simulink library "control_lib"  (R2022b)
settings: Solver=ode45  StartTime=0.0  StopTime=10.0  RelTol=1e-3
settings Model: Creator=nicholas  LastModifiedBy=bensweet
settings SolverCC: AlgebraicLoopSolver=TrustRegion
settings DataIOCC: LimitDataPoints=on  SaveFormat=Array  SignalLoggingSaveFormat=ModelDataLogs  ReturnWorkspaceOutputs=off
settings OptimizationCC: BlockReduction=off  BooleanDataType=off  ExpressionDepthLimit=2147483647  LifeSpan=inf
settings DebuggingCC: SaveWithParameterizedLinksMsg=none  UnderspecifiedInitializationDetection=Classic  MergeDetectMultiDrivingBlocksExec=none  SignalResolutionControl=TryResolveAllWithWarning  UnconnectedInputMsg=warning  UnconnectedOutputMsg=warning  UnconnectedLineMsg=warning  AllowSymbolicDim=off  StateNameClashWarn=warning  PregeneratedLibrarySubsystemCodeDiagnostic=none  SFUnexpectedBacktrackingDiag=warning  SFNoUnconditionalDefaultTransitionDiag=warning  SFExecutionAtInitializationDiag=none  SFMachineParentedDataDiag=warning  ArithmeticOperatorsInVariantConditions=warning
settings HardwareCC: ProdBitPerPointer=32  ProdBitPerSizeT=32  ProdBitPerPtrDiffT=32  ProdLargestAtomicFloat=None  ProdIntDivRoundTo=Undefined  ProdEndianess=Unspecified  ProdWordSize=32  ProdHWDeviceType=32-bit Generic  TargetUnknown=on
settings ModelReferenceCC: EnableRefExpFcnMdlSchedulingChecks=on  PropagateSignalLabelsOutOfModel=off
settings SFSimCC: SimUseLocalCustomCode=off
settings RTWCC: RTWUseLocalCustomCode=off  DLArmComputeVersion=19.05
settings CodeAppCC: StateflowObjectComments=on
settings GRTTargetCC: TargetLangStandard=C89/C90 (ANSI)
settings ConfigComp: CovMetricSettings=dw  CovSaveCumulativeToWorkspaceVar=on  CovSaveSingleToWorkspaceVar=on  CovExternalEMLEnable=off  CovSFcnEnable=off

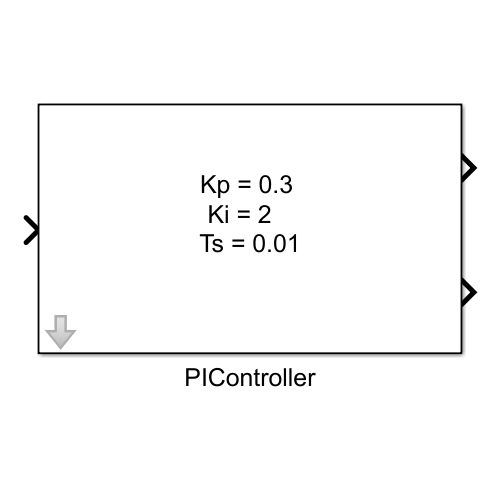
[thumbnail: Simulink's stored preview of the top-level diagram]
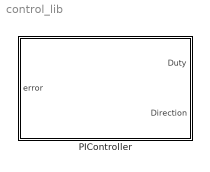
== system control_lib ==
  PIController : Subsystem  mask(PI Controller){Kp=0.3, Ki=2, Ts=0.01}
      mask prompts: Kp "Proportional Gain (Kp)"; Ki "Integral Gain (Ki)"; Ts "Sample Time (Ts)"
      mask help:
      | This system implements the dynamics of a discrete PI controller with a rate limiter on the integrator.
      | You must specify the proportional gain (Kp), integral gain (Ki), and sample time (Ts) for the system.
      mask init:
      | str1 = ['Kp = ',num2str(Kp)];
      | str2 = ['Ki = ',num2str(Ki)];
      | str3 = ['Ts = ',num2str(Ts)];
      | label = strvcat(str1,str2,str3);
      mask Help:
      | This system implements the dynamics of a discrete PI controller with a rate limiter on the integrator.
      | The equations for the system are:  <br /><br />
      | 
      | <b>Y(k) = Yp(k) + Yi(k)</b><br />
      | Yp(k) = Kp*e(k)<br />
      | Yi(k) = Yi(k-1) + Ki*Ts*e(k)<br />
      | -1 < Yi(k) < 1<br /><br />
      | 
      | Define values for Kp, Ki, and Ts for this system.
      mask Display: disp(label)

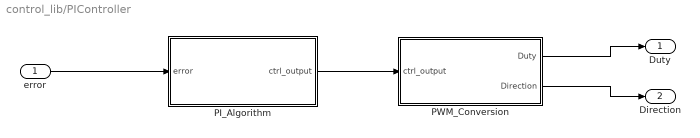
== system control_lib/PIController ==
  error : Inport  SampleTime=Ts
  PI_Algorithm : Subsystem
  PWM_Conversion : Subsystem
  Duty : Outport  VectorParamsAs1DForOutWhenUnconnected=off
  Direction : Outport  Port=2  VectorParamsAs1DForOutWhenUnconnected=off
  wires:
  PI_Algorithm/1(ctrl_output) -> PWM_Conversion/1(ctrl_output)
  PWM_Conversion/2(Direction) -> Direction/1
  PWM_Conversion/1("Duty ") -> Duty/1
  error/1 -> PI_Algorithm/1(error)

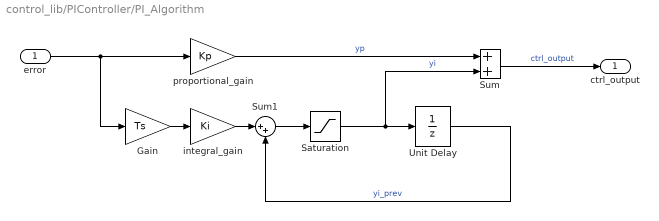
== system control_lib/PIController/PI_Algorithm ==
  error : Inport  SampleTime=Ts
      settings: AttributesFormatString=Sample time = %<SampleTime>
  Gain : Gain  Gain=Ts  SaturateOnIntegerOverflow=on  OutDataTypeStr=Inherit: Same as input  ParamDataTypeStr=Inherit: Same as input
  Saturation : Saturate  UpperLimit=1  LowerLimit=-1
      settings: AttributesFormatString=Max: %<UpperLimit>\nMin: %<LowerLimit>
  Sum : Sum  InputSameDT=on  SaturateOnIntegerOverflow=on  OutDataTypeStr=Inherit: Same as first input
  Sum1 : Sum  Inputs=|++  InputSameDT=on  SaturateOnIntegerOverflow=on  OutDataTypeStr=Inherit: Same as first input
  Unit Delay : UnitDelay  SampleTime=Ts  HasFrameUpgradeWarning=on
      settings: AttributesFormatString=yi0 = %<X0>\nSample time = %<SampleTime>
  integral_gain : Gain  Gain=Ki  SaturateOnIntegerOverflow=on  OutDataTypeStr=Inherit: Same as input  ParamDataTypeStr=Inherit: Same as input
  proportional_gain : Gain  Gain=Kp  SaturateOnIntegerOverflow=on  OutDataTypeStr=Inherit: Same as input  ParamDataTypeStr=Inherit: Same as input
  ctrl_output : Outport  VectorParamsAs1DForOutWhenUnconnected=off
  wires:
  Sum/1 -> ctrl_output/1  "ctrl_output"
  error/1 -> Gain/1, proportional_gain/1
  Saturation/1 -> Sum/2, Unit Delay/1  "yi"
  Sum1/1 -> Saturation/1
  Unit Delay/1 -> Sum1/2  "yi_prev"
  Gain/1 -> integral_gain/1
  integral_gain/1 -> Sum1/1
  proportional_gain/1 -> Sum/1  "yp"

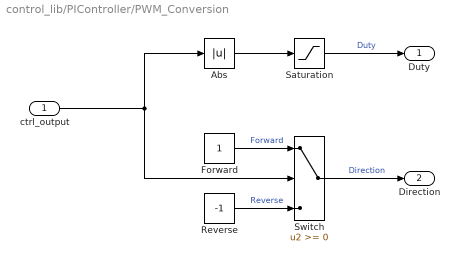
== system control_lib/PIController/PWM_Conversion ==
  ctrl_output : Inport
  Abs : Abs  SaturateOnIntegerOverflow=off
  Forward : Constant  OutDataTypeStr=double
  Reverse : Constant  Value=-1  OutDataTypeStr=double
  Saturation : Saturate  UpperLimit=1  LowerLimit=0
      settings: AttributesFormatString=%<LowerLimit> < duty < %<UpperLimit>
  Switch : Switch  SaturateOnIntegerOverflow=off  InputSameDT=off
      settings: AttributesFormatString=Criteria: %<Criteria>\nThreshold: %<Threshold>
  "Duty " : Outport  VectorParamsAs1DForOutWhenUnconnected=off
  Direction : Outport  Port=2  VectorParamsAs1DForOutWhenUnconnected=off
  wires:
  ctrl_output/1 -> Abs/1, Switch/2
  Forward/1 -> Switch/1  "Forward"
  Reverse/1 -> Switch/3  "Reverse"
  Switch/1 -> Direction/1  "Direction"
  Saturation/1 -> "Duty "/1  "Duty"
  Abs/1 -> Saturation/1
